simulink model "boostconverter"  (R2023b)
settings: Solver=VariableStepAuto  StartTime=0.0  StopTime=10.0  RelTol=1e-3
libraries: spsSeriesRLCBranchLib x3, spsDiodeLib x1, spsMosfetLib x1, spsPWMGeneratorDCDCLib x1, spsDCVoltageSourceLib x1, spsVoltageMeasurementLib x1, sps_lib x1
settings Model: Creator=monica  LastModifiedBy=monica

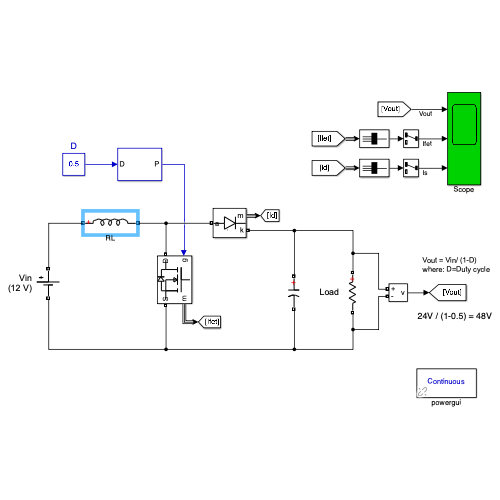
[thumbnail: Simulink's stored preview of the top-level diagram]
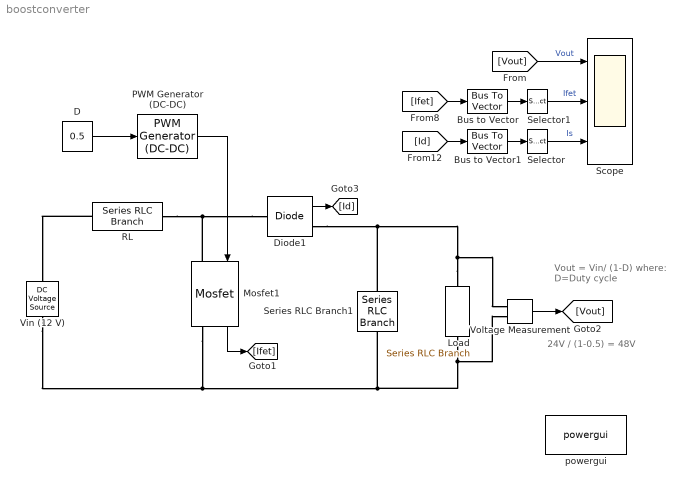
== system boostconverter ==
  note: 24V / (1-0.5) = 48V
  note: Vout = Vin/ (1-D)
      | where: D=Duty cycle
  Bus to Vector : BusToVector
  Bus to Vector1 : BusToVector
  D : Constant  Value=0.5
  Diode1 : spsDiodeLib/Diode  Ron=1e-3  Lon=0  Vf=0  IC=0  UseSnubber=off  Rs=inf  Cs=inf  Measurements=on
  Load : spsSeriesRLCBranchLib/Series RLC Branch  LConnTagsString=__new0  RConnTagsString=__new0  BranchType=R  Resistance=3  Inductance=200e-6  SetiL0=off  InitialCurrent=0  Capacitance=400e-6  Setx0=off  InitialVoltage=0  Measurements=None
  Mosfet1 : spsMosfetLib/Mosfet  Ron=1e-3  Lon=0  Rd=1e-3  Vfd=0  IC=0  Rs=inf  Cs=inf  Measurements=on
  PWM Generator (DC-DC) : spsPWMGeneratorDCDCLib/PWM Generator (DC-DC)  Fsw=20e3  Ts=0
  RL : spsSeriesRLCBranchLib/Series RLC Branch  LConnTagsString=__new0  RConnTagsString=__new0  BranchType=L  Resistance=1e-3  Inductance=4e-6  SetiL0=off  InitialCurrent=0  Capacitance=1e-6  Setx0=off  InitialVoltage=0  Measurements=None
  Scope : Scope  NumInputPorts=3
  Selector : Selector  InputPortWidth=2  IndexOptions=Index vector (dialog)  Indices=1  OutputSizes=1
  Selector1 : Selector  InputPortWidth=2  IndexOptions=Index vector (dialog)  Indices=1  OutputSizes=1
  Series RLC Branch1 : spsSeriesRLCBranchLib/Series RLC Branch  LConnTagsString=__new0  RConnTagsString=__new0  BranchType=C  Resistance=1e-4  Inductance=200e-6  SetiL0=off  InitialCurrent=0  Capacitance=200e-6  Setx0=off  InitialVoltage=40  Measurements=None
  Vin (12 V) : spsDCVoltageSourceLib/DC Voltage Source  Amplitude=12  Measurements=None
  Voltage Measurement : spsVoltageMeasurementLib/Voltage Measurement  PhasorSimulation=off  OutputType=Complex  PSBequivalent=0
  powergui : sps_lib/powergui  Priority=1  SimulationMode=Continuous  SampleTime=50e-6  frequency=60  Iterations=50  frequencyindice=0  Pbase=100e6  ErrMax=1e-4  UnitsV=kV  UnitsW=MW  buscounter=0  FunctionMessages=off  echomessages=off  EnableUseOfTLC=off  CurrentSourceSwitches=off  DisableSnubberDevices=off  DisableRonSwitches=off  DisableVfSwitches=off  DisplayEquations=off  AutomaticDiscreteSolvers=off  SolverType=Tustin/Backward Euler (TBE)  Interpol=off  ExternalGateDelay=off  methode=off  Ts=100  x0status=blocks  SPID=on  SwTol=0  HookPort=off  NonlinearTolerance=1e-4  nMaxIteration=100  ContinueOnMaxIteration=off  RestoreLinks=warning  ResistiveCurrentMeasurement=off  Frange=[0:2:500]  Ylog=off  Xlog=on  ShowGrid=off  save=off  variable=ZData  structure=0  ZoomFFT=off  StartTime=0.0  cycles=1  DisplayStyle=1  fundamental=60  FreqAxis=off  MaxFrequency=1000  frequencyindicesteady=1  RmsSteady=1  display=off
  wires:
  Bus to Vector1/1 -> Selector/1
  PWM Generator (DC-DC)/1 -> Mosfet1/1
  Mosfet1/1 -> [Ifet]
  [Id] -> Bus to Vector1/1
  [Vout] -> Scope/1  "Vout"
  Selector/1 -> Scope/3  "Is"
  [Ifet] -> Bus to Vector/1
  Diode1/1 -> [Id]
  Selector1/1 -> Scope/2  "Ifet"
  D/1 -> PWM Generator (DC-DC)/1
  Bus to Vector/1 -> Selector1/1
  Voltage Measurement/1 -> [Vout]
  connections:
  Series RLC Branch1/RConn1 -- Load/RConn1 -- Voltage Measurement/LConn2 -- Mosfet1/RConn1 -- Vin (12 V)/LConn1
  Load/LConn1 -- Series RLC Branch1/LConn1 -- Diode1/RConn1 -- Voltage Measurement/LConn1
  Diode1/LConn1 -- RL/RConn1 -- Mosfet1/LConn1
  RL/LConn1 -- Vin (12 V)/RConn1
